simulink model "batterycircuitmodel3"  (R2017b)
settings: Solver=ode23tb  StartTime=0.0  StopTime=5  MaxStep=1e-3  RelTol=1e-3
undefined symbols (not defined in the file): Ion, Lithium
libraries: powerlib x23, electricdrivelib x2, powerlib_meascontrol x1
settings Model: Creator=RICHARD MARTIN  LastModifiedBy=RICHARD MARTIN

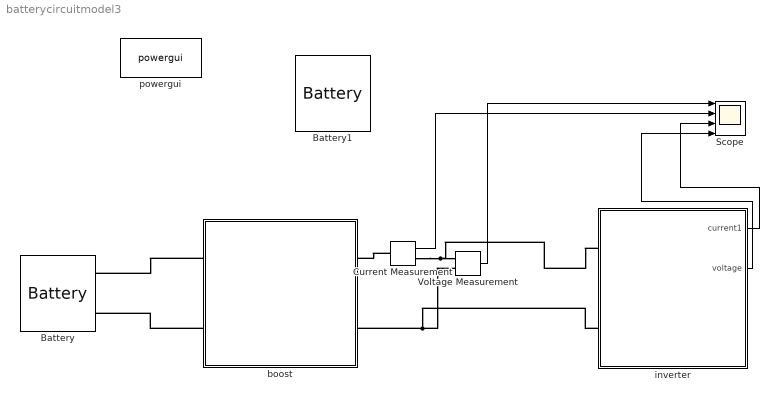
== system batterycircuitmodel3 ==
  Battery : electricdrivelib/Extra Sources/Battery  BatType=Lithium-Ion  ShowTempParam=off  ThermalPreset=no  ShowAgeParam=off  NomV=24  NomQ=16  SOC=95  Batt_Tr=1  PresetModel=off  MaxQ=8  MinV=20  FullV=26  Dis_rate=4  R=0.013333  Normal_OP=8  expZone="[24     8]"  current=[6.5 13 32.5]  Units=Time  Tci=20  NomT=20  T2=-30  MaxQ2=4.8  FullV2=7.1  Normal_OP2=5.655  expZone2="[6.58           1]"  Rca=0.6  ti=2000  Dp=0  Neq0=0  Tsim=1e6  Ta1=25  Qeol=5.4*0.9  Reol=0.013333*1.2  Char_age=[2.3478, 3]  Dis_age=[2.3478, 10]  N1=1500  N2=10500  N3=1000  N4=1400  Ta2=45  N5=950
  Battery1 : electricdrivelib/Extra Sources/Battery  BatType=Lithium-Ion  ShowTempParam=off  ThermalPreset=no  ShowAgeParam=off  NomV=24  NomQ=8  SOC=95  Batt_Tr=1  PresetModel=off  MaxQ=8  MinV=20  FullV=26  Dis_rate=4  R=0.013333  Normal_OP=8  expZone="[24     8]"  current=[6.5 13 32.5]  Units=Time  Tci=20  NomT=20  T2=-30  MaxQ2=4.8  FullV2=7.1  Normal_OP2=5.655  expZone2="[6.58           1]"  Rca=0.6  ti=2000  Dp=0  Neq0=0  Tsim=1e6  Ta1=25  Qeol=5.4*0.9  Reol=0.013333*1.2  Char_age=[2.3478, 3]  Dis_age=[2.3478, 10]  N1=1500  N2=10500  N3=1000  N4=1400  Ta2=45  N5=950
  Current Measurement : powerlib/Measurements/Current Measurement  PhasorSimulation=off  OutputType=Complex  PSBequivalent=0
  Scope : Scope  NumInputPorts=4
  Voltage Measurement : powerlib/Measurements/Voltage Measurement  PhasorSimulation=off  OutputType=Complex  PSBequivalent=0
  boost : Subsystem
  inverter : Subsystem
  powergui : powerlib/powergui  Priority=1  SimulationMode=Continuous  SampleTime=50e-6  frequency=60  Iterations=50  frequencyindice=0  Pbase=100e6  ErrMax=1e-4  UnitsV=kV  UnitsW=MW  buscounter=0  FunctionMessages=off  echomessages=off  EnableUseOfTLC=off  CurrentSourceSwitches=off  DisableSnubberDevices=off  DisableRonSwitches=off  DisableVfSwitches=off  DisplayEquations=off  SolverType=Tustin/Backward Euler (TBE)  Interpol=off  ExternalGateDelay=off  methode=off  Ts=100  x0status=blocks  SPID=on  SwTol=0  HookPort=off  RestoreLinks=warning  ResistiveCurrentMeasurement=off  Frange=[0:2:500]  Ylog=off  Xlog=on  ShowGrid=off  save=off  variable=ZData  structure=0  ZoomFFT=off  StartTime=0.0  cycles=1  DisplayStyle=1  fundamental=60  FreqAxis=off  MaxFrequency=1000  frequencyindicesteady=1  RmsSteady=1  display=off
  wires:
  Voltage Measurement/1 -> Scope/1
  inverter/1(current1) -> Scope/3
  inverter/2(voltage) -> Scope/4
  Current Measurement/1 -> Scope/2
  connections:
  boost/LConn1 -- Battery/LConn1
  boost/LConn2 -- Battery/LConn2
  Voltage Measurement/LConn2 -- inverter/LConn2 -- boost/RConn2
  Current Measurement/LConn1 -- boost/RConn1
  Current Measurement/RConn1 -- inverter/LConn1 -- Voltage Measurement/LConn1

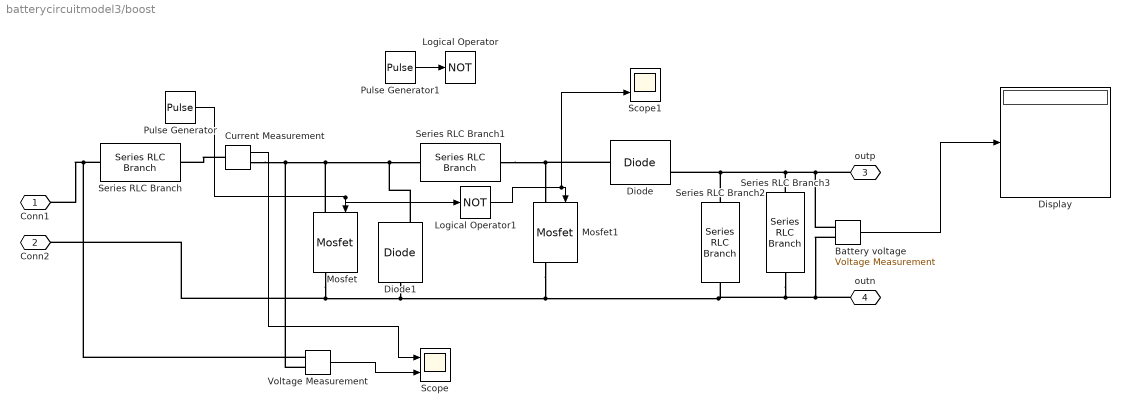
== system batterycircuitmodel3/boost ==
  " Battery voltage " : powerlib/Measurements/Voltage Measurement  PhasorSimulation=off  OutputType=Complex  PSBequivalent=0
  Current Measurement : powerlib/Measurements/Current Measurement  PhasorSimulation=off  OutputType=Complex  PSBequivalent=0
  Diode : powerlib/Power Electronics/Diode  Ron=0.001  Lon=0  Vf=0.8  IC=0  UseSnubber=0  Rs=500  Cs=250e-9  Measurements=on
  Diode1 : powerlib/Power Electronics/Diode  Ron=0.001  Lon=0  Vf=0.8  IC=0  UseSnubber=0  Rs=500  Cs=250e-9  Measurements=on
  Display : Display
  Logical Operator : Logic  Operator=NOT  AllPortsSameDT=off  OutDataTypeStr=boolean
  Logical Operator1 : Logic  Operator=NOT  AllPortsSameDT=off  OutDataTypeStr=boolean
  Mosfet : powerlib/Power Electronics/Mosfet  Ron=0.1  Lon=0  Rd=0.01  Vfd=0  IC=0  Rs=1e5  Cs=inf  Measurements=on
  Mosfet1 : powerlib/Power Electronics/Mosfet  Ron=0.1  Lon=0  Rd=0.01  Vfd=0  IC=0  Rs=1e5  Cs=inf  Measurements=on
  Pulse Generator : DiscretePulseGenerator  PulseType=Time based  Period=0.04e-3  PulseWidth=25
  Pulse Generator1 : DiscretePulseGenerator  PulseType=Time based  Period=0.04e-3  PulseWidth=35
  Scope : Scope  NumInputPorts=2
  Scope1 : Scope  NumInputPorts=2
  Series RLC Branch : powerlib/Elements/Series RLC Branch  LConnTagsString=__new0  RConnTagsString=__new0  BranchType=L  Resistance=1  Inductance=7.3e-3  SetiL0=off  InitialCurrent=0  Capacitance=1e-6  Setx0=off  InitialVoltage=0  Measurements=None
  Series RLC Branch1 : powerlib/Elements/Series RLC Branch  LConnTagsString=__new0  RConnTagsString=__new0  BranchType=L  Resistance=1  Inductance=14.6e-3  SetiL0=off  InitialCurrent=0  Capacitance=1e-6  Setx0=off  InitialVoltage=0  Measurements=None
  Series RLC Branch2 : powerlib/Elements/Series RLC Branch  LConnTagsString=__new0  RConnTagsString=__new0  BranchType=C  Resistance=1  Inductance=1e-3  SetiL0=off  InitialCurrent=0  Capacitance=1000e-3  Setx0=off  InitialVoltage=0  Measurements=None
  Series RLC Branch3 : powerlib/Elements/Series RLC Branch  LConnTagsString=__new0  RConnTagsString=__new0  BranchType=R  Resistance=1e3  Inductance=1e-3  SetiL0=off  InitialCurrent=0  Capacitance=100e-6  Setx0=off  InitialVoltage=0  Measurements=None
  Voltage Measurement : powerlib/Measurements/Voltage Measurement  PhasorSimulation=off  OutputType=Complex  PSBequivalent=0
  Conn1 : PMIOPort  Port=1  Side=Left
  Conn2 : PMIOPort  Port=2  Side=Left
  outp : PMIOPort  Port=3  Side=Right
  outn : PMIOPort  Port=4  Side=Right
  wires:
  Pulse Generator1/1 -> Logical Operator/1
  Voltage Measurement/1 -> Scope/2
  Current Measurement/1 -> Scope/1
  Logical Operator1/1 -> Scope1/2, Mosfet1/1
  " Battery voltage "/1 -> Display/1
  Pulse Generator/1 -> Logical Operator1/1, Mosfet/1
  connections:
  outp/RConn1 -- " Battery voltage "/LConn1 -- Series RLC Branch3/LConn1 -- Series RLC Branch2/LConn1 -- Diode/RConn1
  Diode/LConn1 -- Mosfet1/LConn1 -- Series RLC Branch1/RConn1
  Series RLC Branch/LConn1 -- Voltage Measurement/LConn1 -- Conn1/RConn1
  Mosfet/LConn1 -- Voltage Measurement/LConn2 -- Current Measurement/RConn1 -- Diode1/RConn1 -- Series RLC Branch1/LConn1
  Series RLC Branch2/RConn1 -- outn/RConn1 -- " Battery voltage "/LConn2 -- Series RLC Branch3/RConn1 -- Diode1/LConn1 -- Conn2/RConn1 -- Mosfet/RConn1 -- Mosfet1/RConn1
  Current Measurement/LConn1 -- Series RLC Branch/RConn1

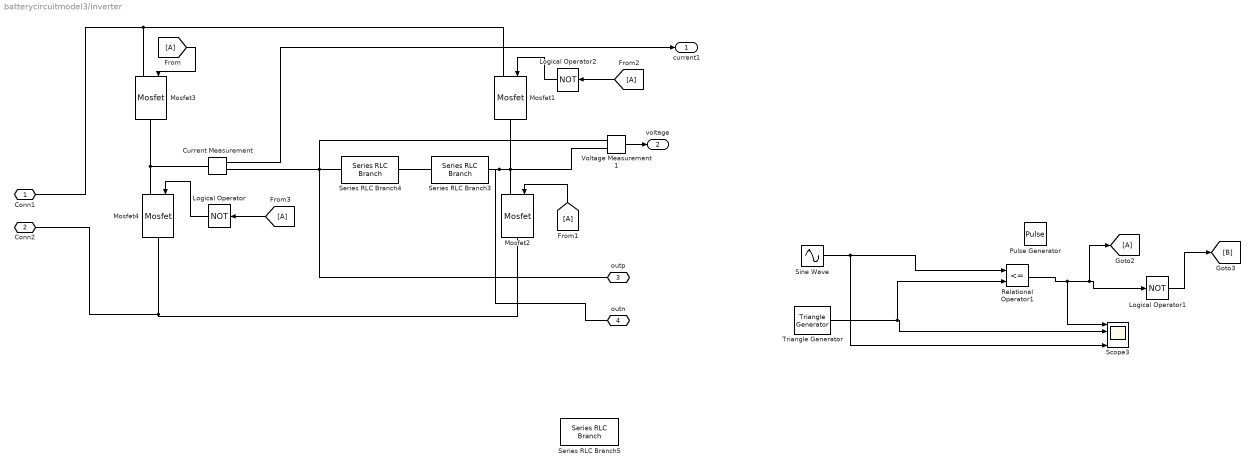
== system batterycircuitmodel3/inverter ==
  Current Measurement : powerlib/Measurements/Current Measurement  PhasorSimulation=off  OutputType=Complex  PSBequivalent=0
  Logical Operator : Logic  Operator=NOT  AllPortsSameDT=off  OutDataTypeStr=boolean
  Logical Operator1 : Logic  Operator=NOT  AllPortsSameDT=off  OutDataTypeStr=boolean
  Logical Operator2 : Logic  Operator=NOT  AllPortsSameDT=off  OutDataTypeStr=boolean
  Mosfet{1..4} (4 alike) : powerlib/Power Electronics/Mosfet  Ron=0.1  Lon=0  Rd=0.01  Vfd=0  IC=0  Rs=1e5  Cs=inf  Measurements=off
  Pulse Generator : DiscretePulseGenerator  PulseType=Time based  Period=.02  PulseWidth=50
  Relational Operator1 : RelationalOperator  Operator=<=  OutDataTypeStr=boolean  RndMeth=Simplest
  Scope3 : Scope  NumInputPorts=4
  Series RLC Branch3 : powerlib/Elements/Series RLC Branch  LConnTagsString=__new0  RConnTagsString=__new0  BranchType=R  Resistance=100  Inductance=1e-3  SetiL0=off  InitialCurrent=0  Capacitance=1e-6  Setx0=off  InitialVoltage=0  Measurements=None
  Series RLC Branch4 : powerlib/Elements/Series RLC Branch  LConnTagsString=__new0  RConnTagsString=__new0  BranchType=L  Resistance=100  Inductance=1e-3  SetiL0=off  InitialCurrent=0  Capacitance=1e-6  Setx0=off  InitialVoltage=0  Measurements=None
  Series RLC Branch5 : powerlib/Elements/Series RLC Branch  LConnTagsString=__new0  RConnTagsString=__new0  BranchType=C  Resistance=100  Inductance=350e-3  SetiL0=off  InitialCurrent=0  Capacitance=10e-6  Setx0=off  InitialVoltage=0  Measurements=None
  Sine Wave : Sin  Amplitude=0.9  Frequency=50*2*pi  SampleTime=0
  Triangle Generator : powerlib_meascontrol/Pulse & Signal Generators/Triangle Generator  Freq=25e3  Phase=0  Ts=0
  Voltage Measurement1 : powerlib/Measurements/Voltage Measurement  PhasorSimulation=off  OutputType=Complex  PSBequivalent=0
  Conn1 : PMIOPort  Port=1  Side=Left
  Conn2 : PMIOPort  Port=2  Side=Left
  outp : PMIOPort  Port=3  Side=Right
  outn : PMIOPort  Port=4  Side=Right
  current1 : Outport
  voltage : Outport  Port=2
  wires:
  Voltage Measurement1/1 -> voltage/1
  Current Measurement/1 -> current1/1
  [A] -> Mosfet2/1
  [A] -> Mosfet3/1
  Relational Operator1/1 -> Scope3/1, [A], Logical Operator1/1
  Sine Wave/1 -> Scope3/4, Relational Operator1/1
  Triangle Generator/1 -> Relational Operator1/2, Scope3/2
  Logical Operator1/1 -> [B]
  Logical Operator/1 -> Mosfet4/1
  [A] -> Logical Operator/1
  Logical Operator2/1 -> Mosfet1/1
  [A] -> Logical Operator2/1
  connections:
  Mosfet2/RConn1 -- Mosfet4/RConn1 -- Conn2/RConn1
  Series RLC Branch3/RConn1 -- Voltage Measurement1/LConn2 -- Mosfet1/RConn1 -- Mosfet2/LConn1 -- outn/RConn1
  Current Measurement/LConn1 -- Mosfet4/LConn1 -- Mosfet3/RConn1
  Voltage Measurement1/LConn1 -- Series RLC Branch4/LConn1 -- outp/RConn1 -- Current Measurement/RConn1
  Mosfet1/LConn1 -- Mosfet3/LConn1 -- Conn1/RConn1
  Series RLC Branch4/RConn1 -- Series RLC Branch3/LConn1
